simulink model "DS_distrIntp_4_0_realaxes"  (R2019b)
settings: Solver=FixedStepDiscrete  StartTime=0.0  StopTime=inf  FixedStep=Ts  RelTol=1e-3
StartFcn:
  | close all;
model workspace (MAT data in the model file):
  MvmtPerfEval_collectVal : Simulink.Parameter (value not decoded)
  MvmtPerfEval_sendOwnVal : Simulink.Parameter (value not decoded)
  PAR_center_c2 : Simulink.Parameter (value not decoded)
  PAR_numStepsAheadSmoothing : Simulink.Parameter (value not decoded)
  PAR_startPosReachedTol : Simulink.Parameter (value not decoded)
  PAR_workspace_c2 : Simulink.Parameter (value not decoded)
  PerfEval_numTicks_enable : Simulink.Parameter (value not decoded)
  Segmentregler_I_Gain : Simulink.Parameter (value not decoded)
  Segmentregler_P_Gain : Simulink.Parameter (value not decoded)
  Segmentregler_minVel_enable : Simulink.Parameter (value not decoded)
  Segmentregler_numTicks_enable : Simulink.Parameter (value not decoded)
  Ts : Simulink.Parameter (value not decoded)
  horizon : Simulink.Parameter (value not decoded)
  maxPos_x : Simulink.Parameter (value not decoded)
  maxPos_y : Simulink.Parameter (value not decoded)
  maxPos_z : Simulink.Parameter (value not decoded)
  maxVectorLengths : Simulink.Parameter (value not decoded)
  minAllowedVelSaturation : Simulink.Parameter (value not decoded)
  numAxes : Simulink.Parameter (value not decoded)
  window_length : Simulink.Parameter (value not decoded)
symbols that are objects in the model workspace (value not decoded): MvmtPerfEval_collectVal, MvmtPerfEval_sendOwnVal, numAxes, PAR_center_c2, PAR_numStepsAheadSmoothing, PAR_startPosReachedTol, PAR_workspace_c2, Ts
undefined symbols (not defined in the file or in its folder): DiscIntNeverNeededParam, setP_mat, VelOverride
libraries: vrlib x1, sldrtlib x1
(part 3 of 4)

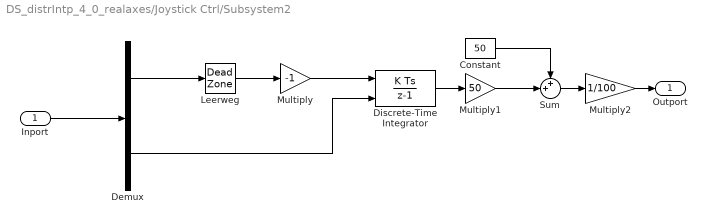
== system DS_distrIntp_4_0_realaxes/Joystick Ctrl/Subsystem2 ==
  Inport : Inport
  Constant : Constant  Value=50
  Demux : Demux  Outputs=2
  Discrete-Time Integrator : DiscreteIntegrator  gainval=0.5  ExternalReset=rising  SampleTime=-1  LimitOutput=on  UpperSaturationLimit=1  LowerSaturationLimit=-0.9  ICPrevOutput=DiscIntNeverNeededParam  ICPrevScaledInput=DiscIntNeverNeededParam
  Leerweg : DeadZone  LowerValue=-0.3  UpperValue=0.3  SaturateOnIntegerOverflow=on
  Multiply : Gain  Gain=-1
  Multiply1 : Gain  Gain=50
  Multiply2 : Gain  Gain=1/100
  Sum : Sum  Inputs=++|
  Outport : Outport  VectorParamsAs1DForOutWhenUnconnected=off
  wires:
  Multiply2/1 -> Outport/1
  Demux/2 -> Discrete-Time Integrator/2
  Demux/1 -> Leerweg/1
  Inport/1 -> Demux/1
  Sum/1 -> Multiply2/1
  Multiply1/1 -> Sum/2
  Multiply/1 -> Discrete-Time Integrator/1
  Discrete-Time Integrator/1 -> Multiply1/1
  Constant/1 -> Sum/1
  Leerweg/1 -> Multiply/1

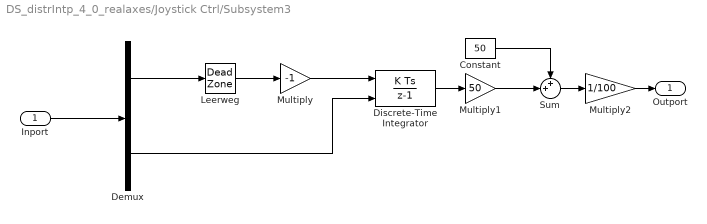
== system DS_distrIntp_4_0_realaxes/Joystick Ctrl/Subsystem3 ==
  Inport : Inport
  Constant : Constant  Value=50
  Demux : Demux  Outputs=2
  Discrete-Time Integrator : DiscreteIntegrator  gainval=0.5  ExternalReset=rising  SampleTime=-1  LimitOutput=on  UpperSaturationLimit=1  LowerSaturationLimit=-0.9  ICPrevOutput=DiscIntNeverNeededParam  ICPrevScaledInput=DiscIntNeverNeededParam
  Leerweg : DeadZone  LowerValue=-0.3  UpperValue=0.3  SaturateOnIntegerOverflow=on
  Multiply : Gain  Gain=-1
  Multiply1 : Gain  Gain=50
  Multiply2 : Gain  Gain=1/100
  Sum : Sum  Inputs=++|
  Outport : Outport  VectorParamsAs1DForOutWhenUnconnected=off
  wires:
  Leerweg/1 -> Multiply/1
  Constant/1 -> Sum/1
  Discrete-Time Integrator/1 -> Multiply1/1
  Multiply/1 -> Discrete-Time Integrator/1
  Multiply1/1 -> Sum/2
  Sum/1 -> Multiply2/1
  Inport/1 -> Demux/1
  Demux/1 -> Leerweg/1
  Demux/2 -> Discrete-Time Integrator/2
  Multiply2/1 -> Outport/1

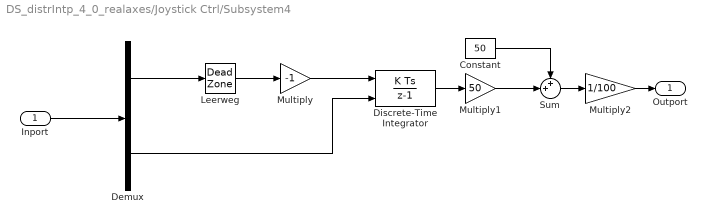
== system DS_distrIntp_4_0_realaxes/Joystick Ctrl/Subsystem4 ==
  Inport : Inport
  Constant : Constant  Value=50
  Demux : Demux  Outputs=2
  Discrete-Time Integrator : DiscreteIntegrator  gainval=0.5  ExternalReset=rising  SampleTime=-1  LimitOutput=on  UpperSaturationLimit=1  LowerSaturationLimit=-0.9  ICPrevOutput=DiscIntNeverNeededParam  ICPrevScaledInput=DiscIntNeverNeededParam
  Leerweg : DeadZone  LowerValue=-0.3  UpperValue=0.3  SaturateOnIntegerOverflow=on
  Multiply : Gain  Gain=-1
  Multiply1 : Gain  Gain=50
  Multiply2 : Gain  Gain=1/100
  Sum : Sum  Inputs=++|
  Outport : Outport  VectorParamsAs1DForOutWhenUnconnected=off
  wires:
  Leerweg/1 -> Multiply/1
  Constant/1 -> Sum/1
  Discrete-Time Integrator/1 -> Multiply1/1
  Multiply/1 -> Discrete-Time Integrator/1
  Multiply1/1 -> Sum/2
  Sum/1 -> Multiply2/1
  Inport/1 -> Demux/1
  Demux/1 -> Leerweg/1
  Demux/2 -> Discrete-Time Integrator/2
  Multiply2/1 -> Outport/1

== stateflow chart DS_distrIntp_4_0_realaxes/Coordination ==
  state funcs [group]
  state Dispatcher [parallel]
    settings: executionOrder=1
    state Idle
    state Registriere_Achse
      entry: num_registeredAxes = ...
      num_registeredAxes + 1;
    state Erhalte_Koordinationsvektor
      entry:
      num_collectedCVectors = ...
      num_collectedCVectors + 1;
      cVectors = [cVectors; cVector_exchange];
      FLAG_canSend_cVector = 1;
    state Distribute_Coordination_Info
      entry:
      FLAG_cVectors_complete = 1;
    state Registriere_Achsen_bereit
      entry:
      num_readyAxes = num_readyAxes + daten;
      if(num_readyAxes == 16)
      FLAG_allAxesReady = true;
      num_readyAxes = 0;
      end
    state axis_run_counter
      entry:
      num_runningAxes = num_runningAxes + daten;
      if num_runningAxes == 16
      FLAG_startButton = false;
      FLAG_axesRunning = true;
      FLAG_allAxesReady = false;
      end
    state axis_stop_counter
      entry:
      num_runningAxes = num_runningAxes - daten;
      if(num_runningAxes == 0)
      FLAG_stopButton = false;
      FLAG_axesRunning = false;
      end
    state DONE
      entry:
      num_doneAxes = num_doneAxes + 1;
      if num_doneAxes == num_registeredAxes
      %FLAG_stopSim = 1;
      end
    state Movement_Performance_Evaluation
      entry:
      while receive(MvmtPerfCoeff)
      if MvmtPerfCoeff.data > MvmtPerf
      MvmtPerf = MvmtPerfCoeff.data;
      end
      if MvmtPerfCoeff.data == -1
      MvmtPerf = 1;
      end
      discard(MvmtPerfCoeff);
      end
    (default) -> Idle
    Idle -> Registriere_Achse [order 1] : registerAxis
    Registriere_Achse -> Idle
    Idle -> Erhalte_Koordinationsvektor [order 2] : cVector_sent
    Erhalte_Koordinationsvektor -> Idle
    Idle -> Distribute_Coordination_Info [order 3] : [num_collectedCVectors==...
        | num_registeredAxes && ...
        | FLAG_cVectors_complete == 0]
    Distribute_Coordination_Info -> Idle
    Idle -> Registriere_Achsen_bereit [order 4] : axis_ready{daten=axis_ready.data}
    Registriere_Achsen_bereit -> Idle
    Idle -> axis_run_counter [order 5] : axis_isRunning{daten=axis_isRunning.data}
    axis_run_counter -> Idle
    Idle -> axis_stop_counter [order 8] : axis_isNotRunning{daten=axis_isNotRunning.data}
    axis_stop_counter -> Idle
    Idle -> Dispatcher.DONE [order 6] : axis_done
    Dispatcher.DONE -> Idle
    Idle -> Movement_Performance_Evaluation [order 7] : MvmtPerfCoeff
    Movement_Performance_Evaluation -> Idle
  state Axis_X [parallel]
    settings: executionOrder=2
    state Start_Idle
      entry:
      registerAxis.data = true;
      send(registerAxis)
    state Hermite_Interpolation
      entry:
      if FLAG_doAkima == 1
      iP = funcs.DS_hermIntp(setP,setP_dist);
      else
      iP = setP;
      end
    state Koordinationsvektor
      entry:
      cVector_init = funcs.DS_gen_Cvector_init...
      (iP,PAR_isAxis,PAR_maxVel);
    state Koordinationsvektor_austauschen
      during:
      if FLAG_canSend_cVector == 1
      cVector_exchange = cVector_init;
      FLAG_canSend_cVector = 0;
      send(cVector_sent);
      axisHasSentCVector = 1;
      end
      Axis_X.Koordinationsvektor_austauschen -> Axis_X.Koordinationsvektor_austauschen [order 1]
    state Axis_full_reset
      state JogAxis
        entry:
        ResetAxis(PAR_isAxis);
        currPos = GET_istPos(PAR_isAxis,1);
        jogAxis(PAR_isAxis);
      state Check_if_moving
        entry:
        %jogAxis(PAR_isAxis);
        if(abs(currPos - GET_istPos(PAR_isAxis,1)) > ...
        PAR_resetAxis_deltaS)
        axis_is_moving = 1;
        else
        axis_is_moving = 0;
        end
      state Reset_successful
        entry:
        jogAxis(PAR_isAxis);
        axis_is_moving = 0;
        FLAG_resetAxis(PAR_isAxis) = 0;
      (default) -> Axis_X.Axis_full_reset.JogAxis
      Axis_X.Axis_full_reset.JogAxis -> Axis_X.Axis_full_reset.Check_if_moving : after(2,'sec')
      Axis_X.Axis_full_reset.Check_if_moving -> Axis_X.Axis_full_reset.JogAxis [order 2] : [axis_is_moving == 0]
      Axis_X.Axis_full_reset.Check_if_moving -> Axis_X.Axis_full_reset.Reset_successful [order 1] : [axis_is_moving == 1]
    state Wait_for_cVectors
    state Find_Consensus
      entry: execVec = funcs.DS_find_Consensus(iP,cVectors,...
      PAR_execIteratorStepSize,PAR_isAxis);
    state Axis_ok
      state Bootstrap_MotionControl
        state JogAxis
          entry:
          ff = ff + 1;
          FLAG_bootstrap_completed = 0;
          %ResetAxis(PAR_isAxis);
          moveRel(PAR_isAxis,PAR_Bootstrap_deltaS,PAR_maxVel/10);
        state GoToStartPos
          entry:
          goToPos(PAR_isAxis,setP(PAR_isAxis,1)*1000,PAR_maxVel*0.5);
        state Check_StartPos_reached
          during:
          if(abs(GET_istPos(PAR_isAxis,1) - setP(PAR_isAxis,1)) <...
          PAR_startPosReachedTol)
          FLAG_bootstrap_completed = 1;
          end
        state StartPos_reached
          entry:
          %on after(3,sec):
          axis_ready.data = 1;
          send(axis_ready);
        (default) -> Axis_X.Axis_ok.Bootstrap_MotionControl.JogAxis
        Axis_X.Axis_ok.Bootstrap_MotionControl.JogAxis -> Axis_X.Axis_ok.Bootstrap_MotionControl.GoToStartPos : after(1,'sec')
        Axis_X.Axis_ok.Bootstrap_MotionControl.GoToStartPos -> Axis_X.Axis_ok.Bootstrap_MotionControl.Check_StartPos_reached
        Axis_X.Axis_ok.Bootstrap_MotionControl.Check_StartPos_reached -> Axis_X.Axis_ok.Bootstrap_MotionControl.StartPos_reached : after(5,sec)[FLAG_bootstrap_completed == 1]
      state Start_run
        entry:
        axis_isRunning.data = 1;
        send(axis_isRunning);
        RUN_idx = 0;
        RUN_startPos(1,PAR_isAxis) = setP(PAR_isAxis,1);
        RUN_num_steps = size(execVec,2);
        state Send_command
          entry:
          RUN_idx = RUN_idx + 1;
          currCVector = cVectors(:,RUN_idx)' ./ VelOverride';
          currCVal = max(currCVector);
          currOverrideAdaptationFactor = execVec(3,RUN_idx) / currCVal; %individueller neuer Override Faktor für diese Achse
          currStepTimeLength = execVec(3,RUN_idx) / currOverrideAdaptationFactor;
          RUN_pos(1,PAR_isAxis) = execVec(1,RUN_idx);
          RUN_vel(1,PAR_isAxis) = execVec(2,RUN_idx) * currOverrideAdaptationFactor;
          MvmtPerf_accumulatedLagTime = MvmtPerf_accumulatedLagTime + (currStepTimeLength - execVec(3,RUN_idx));
          RUN_time(1,PAR_isAxis) = execVec(4,RUN_idx) + MvmtPerf_accumulatedLagTime; %wird nicht benutzt
          RUN_maxVel(1,PAR_isAxis) = PAR_maxVel;
          RUN_MvmtPerfFeedback(1,PAR_isAxis) = 0; %wird zZt nicht benutzt
        state execute_movement
          state DEVEKOS_Ueberschleifen
            entry:
            currStepTimeLength = currStepTimeLength - PAR_numStepsAheadSmoothing*Ts;
          state idle
            entry:
            MvmtPerfCoeff.data = -1;
            send(MvmtPerfCoeff);
          state getOwnPerfCoeff [commented out]
            entry:
            MvmtPerfCoeff.data = GET_perfIndicator(PAR_isAxis);
            send(MvmtPerfCoeff);
          state getMutualPerformance [commented out]
            entry:
            MvmtPerf_accumulatedLagTime = MvmtPerf_accumulatedLagTime + (MvmtPerf-1) * currStepTimeLength;
            RUN_MvmtPerfFeedback(1,PAR_isAxis) = (MvmtPerf-1) * currStepTimeLength;
            RUN_vel(1,PAR_isAxis) = execVec(2,RUN_idx) / MvmtPerf;
            currStepTimeLength = currStepTimeLength * MvmtPerf;
          (default) -> Axis_X.Axis_ok.Start_run.execute_movement.idle
          Axis_X.Axis_ok.Start_run.execute_movement.idle -> Axis_X.Axis_ok.Start_run.execute_movement.DEVEKOS_Ueberschleifen
          Axis_X.Axis_ok.Start_run.execute_movement.idle -> Axis_X.Axis_ok.Start_run.execute_movement.getOwnPerfCoeff [commented out] : after(currStepTimeLength * MvmtPerfEval_sendOwnVal,sec)
          Axis_X.Axis_ok.Start_run.execute_movement.getOwnPerfCoeff -> Axis_X.Axis_ok.Start_run.execute_movement.getMutualPerformance [commented out] : after(currStepTimeLength * (MvmtPerfEval_collectVal - MvmtPerfEval_sendOwnVal),sec)
        (default) -> Axis_X.Axis_ok.Start_run.Send_command
        (junction 638) -> Axis_X.Axis_ok.Start_run.Send_command [order 2]
        Axis_X.Axis_ok.Start_run.Send_command -> Axis_X.Axis_ok.Start_run.execute_movement
        Axis_X.Axis_ok.Start_run.execute_movement -> (junction 638) : after(currStepTimeLength,sec)
      (junction 2099) -> (junction 1942)
      (junction 1947) -> (junction 2099)
      (junction 1942) -> Axis_X.Axis_ok.Bootstrap_MotionControl
      Axis_X.Axis_ok.Bootstrap_MotionControl -> Axis_X.Axis_ok.Start_run [order 2] : [FLAG_allAxesReady == 1 &&...
          |  FLAG_startButton == 1]
      Axis_X.Axis_ok.Bootstrap_MotionControl -> Axis_X.Axis_ok.Start_run [order 1] : [FLAG_allAxesReady == 1 &&...
          |  FLAG_runContinuously == 1]
      Axis_X.Axis_ok.Start_run -> (junction 1947) : [FLAG_stopButton == 1]...
          | {StopAxis(PAR_isAxis);...
          | axis_isNotRunning.data = 1;...
          | send(axis_isNotRunning)}
    state DONE
      entry:
      StopAxis(PAR_isAxis);
      %send(axis_isNotRunning);
      %send(axis_done);
      exit:
      axis_isNotRunning.data = 1;
      send(axis_isNotRunning);
    (default) -> Axis_X.Start_Idle
    Axis_X.Start_Idle -> Axis_X.Hermite_Interpolation
    Axis_X.Hermite_Interpolation -> Axis_X.Koordinationsvektor
    Axis_X.Koordinationsvektor -> Axis_X.Koordinationsvektor_austauschen
    Axis_X.Koordinationsvektor_austauschen -> Axis_X.Wait_for_cVectors [order 1] : [axisHasSentCVector == 1]
    Axis_X.Wait_for_cVectors -> Axis_X.Find_Consensus : [FLAG_cVectors_complete == 1]
    Axis_X.Axis_full_reset -> (junction 2110) : [FLAG_resetAxis(PAR_isAxis) == 0]
    Axis_X.Axis_ok -> Axis_X.Axis_full_reset : [FLAG_resetAxis(PAR_isAxis) == 1]...
        | {StopAxis(PAR_isAxis);...
        | axis_isNotRunning.data = 1;...
        | send(axis_isNotRunning)}
    Axis_X.Find_Consensus -> (junction 2103)
    (junction 2110) -> (junction 2103)
    (junction 2103) -> (junction 1942)
    (junction 2388) -> (junction 1947)
    (junction 638) -> Axis_X.DONE [order 1] : [RUN_idx == RUN_num_steps]
    Axis_X.DONE -> (junction 2388)
  state Axis_Y [parallel]
    settings: executionOrder=3
    state Start_Idle
      entry:
      registerAxis.data = true;
      send(registerAxis)
    state Hermite_Interpolation
      entry:
      if FLAG_doAkima == 1
      iP = funcs.DS_hermIntp(setP,setP_dist);
      else
      iP = setP;
      end
    state Koordinationsvektor
      entry:
      cVector_init = funcs.DS_gen_Cvector_init...
      (iP,PAR_isAxis,PAR_maxVel);
    state Koordinationsvektor_austauschen
      during:
      if FLAG_canSend_cVector == 1
      cVector_exchange = cVector_init;
      FLAG_canSend_cVector = 0;
      send(cVector_sent);
      axisHasSentCVector = 1;
      end
      Axis_Y.Koordinationsvektor_austauschen -> Axis_Y.Koordinationsvektor_austauschen [order 1]
    state Axis_full_reset
      state JogAxis
        entry:
        ResetAxis(PAR_isAxis);
        currPos = GET_istPos(PAR_isAxis,1);
        jogAxis(PAR_isAxis);
      state Check_if_moving
        entry:
        %jogAxis(PAR_isAxis);
        if(abs(currPos - GET_istPos(PAR_isAxis,1)) > ...
        PAR_resetAxis_deltaS)
        axis_is_moving = 1;
        else
        axis_is_moving = 0;
        end
      state Reset_successful
        entry:
        jogAxis(PAR_isAxis);
        axis_is_moving = 0;
        FLAG_resetAxis(PAR_isAxis) = 0;
      (default) -> Axis_Y.Axis_full_reset.JogAxis
      Axis_Y.Axis_full_reset.JogAxis -> Axis_Y.Axis_full_reset.Check_if_moving : after(2,'sec')
      Axis_Y.Axis_full_reset.Check_if_moving -> Axis_Y.Axis_full_reset.JogAxis [order 2] : [axis_is_moving == 0]
      Axis_Y.Axis_full_reset.Check_if_moving -> Axis_Y.Axis_full_reset.Reset_successful [order 1] : [axis_is_moving == 1]
    state Wait_for_cVectors
    state Find_Consensus
      entry: execVec = funcs.DS_find_Consensus(iP,cVectors,...
      PAR_execIteratorStepSize,PAR_isAxis);
      ff = 1;
    state Axis_ok
      state Bootstrap_MotionControl
        state JogAxis
          entry:
          FLAG_bootstrap_completed = 0;
          ResetAxis(PAR_isAxis);
          moveRel(PAR_isAxis,PAR_Bootstrap_deltaS,PAR_maxVel/10);
        state GoToStartPos
          entry:
          goToPos(PAR_isAxis,setP(PAR_isAxis,1)*1000,PAR_maxVel*0.5);
        state Check_StartPos_reached
          during:
          if(abs(GET_istPos(PAR_isAxis,1) - setP(PAR_isAxis,1)) <...
          PAR_startPosReachedTol)
          FLAG_bootstrap_completed = 1;
          end
        state StartPos_reached
          entry:
          %on after(3,sec):
          axis_ready.data = 3;
          send(axis_ready);
        (default) -> Axis_Y.Axis_ok.Bootstrap_MotionControl.JogAxis
        Axis_Y.Axis_ok.Bootstrap_MotionControl.JogAxis -> Axis_Y.Axis_ok.Bootstrap_MotionControl.GoToStartPos : after(1,'sec')
        Axis_Y.Axis_ok.Bootstrap_MotionControl.GoToStartPos -> Axis_Y.Axis_ok.Bootstrap_MotionControl.Check_StartPos_reached
        Axis_Y.Axis_ok.Bootstrap_MotionControl.Check_StartPos_reached -> Axis_Y.Axis_ok.Bootstrap_MotionControl.StartPos_reached : [FLAG_bootstrap_completed == 1]
      state Start_run
        entry:
        axis_isRunning.data = 3;
        send(axis_isRunning);
        RUN_idx = 0;
        RUN_startPos(1,PAR_isAxis) = setP(PAR_isAxis,1);
        RUN_num_steps = size(execVec,2);
        state Send_command
          entry:
          RUN_idx = RUN_idx + 1;
          currCVector = cVectors(:,RUN_idx)' ./ VelOverride';
          currCVal = max(currCVector);
          currOverrideAdaptationFactor = execVec(3,RUN_idx) / currCVal; %individueller neuer Override Faktor für diese Achse
          currStepTimeLength = execVec(3,RUN_idx) / currOverrideAdaptationFactor;
          RUN_pos(1,PAR_isAxis) = execVec(1,RUN_idx);
          RUN_vel(1,PAR_isAxis) = execVec(2,RUN_idx) * currOverrideAdaptationFactor;
          MvmtPerf_accumulatedLagTime = MvmtPerf_accumulatedLagTime + (currStepTimeLength - execVec(3,RUN_idx));
          RUN_time(1,PAR_isAxis) = execVec(4,RUN_idx) + MvmtPerf_accumulatedLagTime; %wird nicht benutzt
          RUN_maxVel(1,PAR_isAxis) = PAR_maxVel;
          RUN_MvmtPerfFeedback(1,PAR_isAxis) = 0; %wird zZt nicht benutzt
        state execute_movement
          state DEVEKOS_Ueberschleifen
            entry:
            currStepTimeLength = currStepTimeLength - PAR_numStepsAheadSmoothing*Ts;
          state idle
            entry:
            MvmtPerfCoeff.data = -1;
            send(MvmtPerfCoeff);
          state getOwnPerfCoeff [commented out]
            entry:
            MvmtPerfCoeff.data = GET_perfIndicator(PAR_isAxis);
            send(MvmtPerfCoeff);
          state getMutualPerformance [commented out]
            entry:
            MvmtPerf_accumulatedLagTime = MvmtPerf_accumulatedLagTime + (MvmtPerf-1) * currStepTimeLength;
            RUN_MvmtPerfFeedback(1,PAR_isAxis) = (MvmtPerf-1) * currStepTimeLength;
            RUN_vel(1,PAR_isAxis) = execVec(2,RUN_idx) / MvmtPerf;
            currStepTimeLength = currStepTimeLength * MvmtPerf;
          (default) -> Axis_Y.Axis_ok.Start_run.execute_movement.idle
          Axis_Y.Axis_ok.Start_run.execute_movement.idle -> Axis_Y.Axis_ok.Start_run.execute_movement.DEVEKOS_Ueberschleifen
          Axis_Y.Axis_ok.Start_run.execute_movement.idle -> Axis_Y.Axis_ok.Start_run.execute_movement.getOwnPerfCoeff [commented out] : after(currStepTimeLength * MvmtPerfEval_sendOwnVal,sec)
          Axis_Y.Axis_ok.Start_run.execute_movement.getOwnPerfCoeff -> Axis_Y.Axis_ok.Start_run.execute_movement.getMutualPerformance [commented out] : after(currStepTimeLength * (MvmtPerfEval_collectVal - MvmtPerfEval_sendOwnVal),sec)
        (default) -> Axis_Y.Axis_ok.Start_run.Send_command
        (junction 2720) -> Axis_Y.Axis_ok.Start_run.Send_command [order 2]
        Axis_Y.Axis_ok.Start_run.Send_command -> Axis_Y.Axis_ok.Start_run.execute_movement
        Axis_Y.Axis_ok.Start_run.execute_movement -> (junction 2720) : after(currStepTimeLength,sec)
      (junction 2700) -> (junction 2699)
      (junction 2701) -> (junction 2700)
      (junction 2699) -> Axis_Y.Axis_ok.Bootstrap_MotionControl
      Axis_Y.Axis_ok.Bootstrap_MotionControl -> Axis_Y.Axis_ok.Start_run [order 2] : [FLAG_allAxesReady == 1 &&...
          |  FLAG_startButton == 1]
      Axis_Y.Axis_ok.Bootstrap_MotionControl -> Axis_Y.Axis_ok.Start_run [order 1] : [FLAG_allAxesReady == 1 &&...
          |  FLAG_runContinuously == 1]
      Axis_Y.Axis_ok.Start_run -> (junction 2701) : [FLAG_stopButton == 1]...
          | {StopAxis(PAR_isAxis);...
          | axis_isNotRunning.data = 3;...
          | send(axis_isNotRunning)}
    state DONE
      entry:
      StopAxis(PAR_isAxis);
      %send(axis_done);
      exit:
      axis_isNotRunning.data = 3;
      send(axis_isNotRunning);
    (default) -> Axis_Y.Start_Idle
    Axis_Y.Start_Idle -> Axis_Y.Hermite_Interpolation
    Axis_Y.Hermite_Interpolation -> Axis_Y.Koordinationsvektor
    Axis_Y.Koordinationsvektor -> Axis_Y.Koordinationsvektor_austauschen
    Axis_Y.Koordinationsvektor_austauschen -> Axis_Y.Wait_for_cVectors [order 1] : [axisHasSentCVector == 1]
    Axis_Y.Wait_for_cVectors -> Axis_Y.Find_Consensus : [FLAG_cVectors_complete == 1]
    Axis_Y.Axis_full_reset -> (junction 2651) : [FLAG_resetAxis(PAR_isAxis) == 0]
    Axis_Y.Axis_ok -> Axis_Y.Axis_full_reset : [FLAG_resetAxis(PAR_isAxis) == 1]...
        | {StopAxis(PAR_isAxis);...
        | axis_isNotRunning.data = 3;...
        | send(axis_isNotRunning)}
    Axis_Y.Find_Consensus -> (junction 2650)
    (junction 2651) -> (junction 2650)
    (junction 2650) -> (junction 2699)
    (junction 2652) -> (junction 2701)
    (junction 2720) -> Axis_Y.DONE [order 1] : [RUN_idx == RUN_num_steps]
    Axis_Y.DONE -> (junction 2652)
  state Axis_Z [parallel]
    settings: executionOrder=4
    state Start_Idle
      entry:
      registerAxis.data = true;
      send(registerAxis)
    state Hermite_Interpolation
      entry:
      if FLAG_doAkima == 1
      iP = funcs.DS_hermIntp(setP,setP_dist);
      else
      iP = setP;
      end
    state Koordinationsvektor
      entry:
      cVector_init = funcs.DS_gen_Cvector_init...
      (iP,PAR_isAxis,PAR_maxVel);
    state Koordinationsvektor_austauschen
      during:
      if FLAG_canSend_cVector == 1
      cVector_exchange = cVector_init;
      FLAG_canSend_cVector = 0;
      send(cVector_sent);
      axisHasSentCVector = 1;
      end
      Axis_Z.Koordinationsvektor_austauschen -> Axis_Z.Koordinationsvektor_austauschen [order 1]
    state Axis_full_reset
      state JogAxis
        entry:
        ResetAxis(PAR_isAxis);
        currPos = GET_istPos(PAR_isAxis,1);
        jogAxis(PAR_isAxis);
      state Check_if_moving
        entry:
        %jogAxis(PAR_isAxis);
        if(abs(currPos - GET_istPos(PAR_isAxis,1)) > ...
        PAR_resetAxis_deltaS)
        axis_is_moving = 1;
        else
        axis_is_moving = 0;
        end
      state Reset_successful
        entry:
        jogAxis(PAR_isAxis);
        axis_is_moving = 0;
        FLAG_resetAxis(PAR_isAxis) = 0;
      (default) -> Axis_Z.Axis_full_reset.JogAxis
      Axis_Z.Axis_full_reset.JogAxis -> Axis_Z.Axis_full_reset.Check_if_moving : after(2,'sec')
      Axis_Z.Axis_full_reset.Check_if_moving -> Axis_Z.Axis_full_reset.JogAxis [order 2] : [axis_is_moving == 0]
      Axis_Z.Axis_full_reset.Check_if_moving -> Axis_Z.Axis_full_reset.Reset_successful [order 1] : [axis_is_moving == 1]
    state Wait_for_cVectors
    state Find_Consensus
      entry: execVec = funcs.DS_find_Consensus(iP,cVectors,...
      PAR_execIteratorStepSize,PAR_isAxis);
    state Axis_ok
      state Bootstrap_MotionControl
        state JogAxis
          entry:
          FLAG_bootstrap_completed = 0;
          ResetAxis(PAR_isAxis);
          moveRel(PAR_isAxis,PAR_Bootstrap_deltaS,PAR_maxVel/10);
        state GoToStartPos
          entry:
          goToPos(PAR_isAxis,setP(PAR_isAxis,1)*1000,PAR_maxVel*0.5);
        state Check_StartPos_reached
          during:
          if(abs(GET_istPos(PAR_isAxis,1) - setP(PAR_isAxis,1)) <...
          PAR_startPosReachedTol)
          FLAG_bootstrap_completed = 1;
          end
        state StartPos_reached
          entry:
          axis_ready.data = 5;
          send(axis_ready);
        (default) -> Axis_Z.Axis_ok.Bootstrap_MotionControl.JogAxis
        Axis_Z.Axis_ok.Bootstrap_MotionControl.JogAxis -> Axis_Z.Axis_ok.Bootstrap_MotionControl.GoToStartPos : after(1,'sec')
        Axis_Z.Axis_ok.Bootstrap_MotionControl.GoToStartPos -> Axis_Z.Axis_ok.Bootstrap_MotionControl.Check_StartPos_reached
        Axis_Z.Axis_ok.Bootstrap_MotionControl.Check_StartPos_reached -> Axis_Z.Axis_ok.Bootstrap_MotionControl.StartPos_reached : [FLAG_bootstrap_completed == 1]
      state Start_run
        entry:
        axis_isRunning.data = 5;
        send(axis_isRunning);
        RUN_idx = 0;
        RUN_startPos(1,PAR_isAxis) = setP(PAR_isAxis,1);
        RUN_num_steps = size(execVec,2);
        state Send_command
          entry:
          RUN_idx = RUN_idx + 1;
          currCVector = cVectors(:,RUN_idx)' ./ VelOverride';
          currCVal = max(currCVector);
          currOverrideAdaptationFactor = execVec(3,RUN_idx) / currCVal; %individueller neuer Override Faktor für diese Achse
          currStepTimeLength = execVec(3,RUN_idx) / currOverrideAdaptationFactor;
          RUN_pos(1,PAR_isAxis) = execVec(1,RUN_idx);
          RUN_vel(1,PAR_isAxis) = execVec(2,RUN_idx) * currOverrideAdaptationFactor;
          MvmtPerf_accumulatedLagTime = MvmtPerf_accumulatedLagTime + (currStepTimeLength - execVec(3,RUN_idx));
          RUN_time(1,PAR_isAxis) = execVec(4,RUN_idx) + MvmtPerf_accumulatedLagTime; %wird nicht benutzt
          RUN_maxVel(1,PAR_isAxis) = PAR_maxVel;
          RUN_MvmtPerfFeedback(1,PAR_isAxis) = 0; %wird zZt nicht benutzt
        state execute_movement
          state DEVEKOS_Ueberschleifen
            entry:
            currStepTimeLength = currStepTimeLength - PAR_numStepsAheadSmoothing*Ts;
          state idle
            entry:
            MvmtPerfCoeff.data = -1;
            send(MvmtPerfCoeff);
          state getOwnPerfCoeff [commented out]
            entry:
            MvmtPerfCoeff.data = GET_perfIndicator(PAR_isAxis);
            send(MvmtPerfCoeff);
          state getMutualPerformance [commented out]
            entry:
            MvmtPerf_accumulatedLagTime = MvmtPerf_accumulatedLagTime + (MvmtPerf-1) * currStepTimeLength;
            RUN_MvmtPerfFeedback(1,PAR_isAxis) = (MvmtPerf-1) * currStepTimeLength;
            RUN_vel(1,PAR_isAxis) = execVec(2,RUN_idx) / MvmtPerf;
            currStepTimeLength = currStepTimeLength * MvmtPerf;
          (default) -> Axis_Z.Axis_ok.Start_run.execute_movement.idle
          Axis_Z.Axis_ok.Start_run.execute_movement.idle -> Axis_Z.Axis_ok.Start_run.execute_movement.DEVEKOS_Ueberschleifen
          Axis_Z.Axis_ok.Start_run.execute_movement.idle -> Axis_Z.Axis_ok.Start_run.execute_movement.getOwnPerfCoeff [commented out] : after(currStepTimeLength * MvmtPerfEval_sendOwnVal,sec)
          Axis_Z.Axis_ok.Start_run.execute_movement.getOwnPerfCoeff -> Axis_Z.Axis_ok.Start_run.execute_movement.getMutualPerformance [commented out] : after(currStepTimeLength * (MvmtPerfEval_collectVal - MvmtPerfEval_sendOwnVal),sec)
        (default) -> Axis_Z.Axis_ok.Start_run.Send_command
        (junction 2823) -> Axis_Z.Axis_ok.Start_run.Send_command [order 2]
        Axis_Z.Axis_ok.Start_run.Send_command -> Axis_Z.Axis_ok.Start_run.execute_movement
        Axis_Z.Axis_ok.Start_run.execute_movement -> (junction 2823) : after(currStepTimeLength,sec)
      (junction 2803) -> (junction 2802)
      (junction 2804) -> (junction 2803)
      (junction 2802) -> Axis_Z.Axis_ok.Bootstrap_MotionControl
      Axis_Z.Axis_ok.Bootstrap_MotionControl -> Axis_Z.Axis_ok.Start_run [order 2] : [FLAG_allAxesReady == 1 &&...
          |  FLAG_startButton == 1]
      Axis_Z.Axis_ok.Bootstrap_MotionControl -> Axis_Z.Axis_ok.Start_run [order 1] : [FLAG_allAxesReady == 1 &&...
          |  FLAG_runContinuously == 1]
      Axis_Z.Axis_ok.Start_run -> (junction 2804) : [FLAG_stopButton == 1]...
          | {StopAxis(PAR_isAxis);...
          | axis_isNotRunning.data = 5;...
          | send(axis_isNotRunning)}
    state DONE
      entry:
      StopAxis(PAR_isAxis);
      %send(axis_done);
      exit:
      axis_isNotRunning.data = 5;
      send(axis_isNotRunning);
    (default) -> Axis_Z.Start_Idle
    Axis_Z.Start_Idle -> Axis_Z.Hermite_Interpolation
    Axis_Z.Hermite_Interpolation -> Axis_Z.Koordinationsvektor
    Axis_Z.Koordinationsvektor -> Axis_Z.Koordinationsvektor_austauschen
    Axis_Z.Koordinationsvektor_austauschen -> Axis_Z.Wait_for_cVectors [order 1] : [axisHasSentCVector == 1]
    Axis_Z.Wait_for_cVectors -> Axis_Z.Find_Consensus : [FLAG_cVectors_complete == 1]
    Axis_Z.Axis_full_reset -> (junction 2754) : [FLAG_resetAxis(PAR_isAxis) == 0]
    Axis_Z.Axis_ok -> Axis_Z.Axis_full_reset : [FLAG_resetAxis(PAR_isAxis) == 1]...
        | {StopAxis(PAR_isAxis);...
        | axis_isNotRunning.data = 5;...
        | send(axis_isNotRunning)}
    Axis_Z.Find_Consensus -> (junction 2753)
    (junction 2754) -> (junction 2753)
    (junction 2753) -> (junction 2802)
    (junction 2755) -> (junction 2804)
    (junction 2823) -> Axis_Z.DONE [order 1] : [RUN_idx == RUN_num_steps]
    Axis_Z.DONE -> (junction 2755)
  state Axis_C2 [parallel]
    settings: executionOrder=5
    state Start_Idle
      entry:
      registerAxis.data = true;
      send(registerAxis)
    state Bahnpunkte
      entry:
      if FLAG_doAkima == 1
      iP = funcs.DS_hermIntp(setP,setP_dist);
      else
      iP = setP;
      end
      if PAR_isAxis > 3
      iP = [iP;zeros(PAR_isAxis - size(iP,1), length(iP))];
      iP(PAR_isAxis,:) = funcs.PS_gen_Points_Axis...
      (iP,PAR_center_c2,...
      PAR_workspace_c2,...
      PAR_kindOfAxis);
      end
    state Koordinationsvektor
      entry:
      cVector_init = funcs.DS_gen_Cvector_init...
      (iP,PAR_isAxis,PAR_maxVel);
    state Koordinationsvektor_austauschen
      during:
      if FLAG_canSend_cVector == 1
      cVector_exchange = cVector_init;
      FLAG_canSend_cVector = 0;
      send(cVector_sent);
      axisHasSentCVector = 1;
      end
      Axis_C2.Koordinationsvektor_austauschen -> Axis_C2.Koordinationsvektor_austauschen [order 1]
    state Wait_for_cVectors
    state Find_Consensus
      entry:
      execVec = funcs.DS_find_Consensus(iP,cVectors,...
      PAR_execIteratorStepSize,PAR_isAxis);
      axis_ready.data = 7;
      send(axis_ready);
    state Nullen
      entry:
      homingDauerlauf;
    state Homing_done
      entry:
      axis_ready.data = 7;
      send(axis_ready);
    state Start_run
      entry:
      axis_isRunning.data = 7;
      send(axis_isRunning);
      RUN_idx = 0;
      RUN_startPos(1,PAR_isAxis) = iP(PAR_isAxis,1);
      RUN_num_steps = size(execVec,2);
      state Send_command
        entry:
        RUN_idx = RUN_idx + 1;
        currCVector = cVectors(:,RUN_idx)' ./ VelOverride';
        currCVal = max(currCVector);
        currOverrideAdaptationFactor = execVec(3,RUN_idx) / currCVal; %individueller neuer Override Faktor für diese Achse
        currStepTimeLength = execVec(3,RUN_idx) / currOverrideAdaptationFactor;
        RUN_pos(1,PAR_isAxis) = execVec(1,RUN_idx);
        RUN_vel(1,PAR_isAxis) = execVec(2,RUN_idx) * currOverrideAdaptationFactor;
        MvmtPerf_accumulatedLagTime = MvmtPerf_accumulatedLagTime + (currStepTimeLength - execVec(3,RUN_idx));
        RUN_time(1,PAR_isAxis) = execVec(4,RUN_idx) + MvmtPerf_accumulatedLagTime; %wird nicht benutzt
        RUN_maxVel(1,PAR_isAxis) = PAR_maxVel;
        RUN_MvmtPerfFeedback(1,PAR_isAxis) = 0; %wird zZt nicht benutzt
      state execute_movement
        state DEVEKOS_Ueberschleifen
          entry:
          currStepTimeLength = currStepTimeLength - PAR_numStepsAheadSmoothing*Ts;
        state idle
          entry:
          MvmtPerfCoeff.data = -1;
          send(MvmtPerfCoeff);
        state getOwnPerfCoeff [commented out]
          entry:
          MvmtPerfCoeff.data = GET_perfIndicator(PAR_isAxis);
          send(MvmtPerfCoeff);
        state getMutualPerformance [commented out]
          entry:
          MvmtPerf_accumulatedLagTime = MvmtPerf_accumulatedLagTime + (MvmtPerf-1) * currStepTimeLength;
          RUN_MvmtPerfFeedback(1,PAR_isAxis) = (MvmtPerf-1) * currStepTimeLength;
          RUN_vel(1,PAR_isAxis) = execVec(2,RUN_idx) / MvmtPerf;
          currStepTimeLength = currStepTimeLength * MvmtPerf;
        (default) -> Axis_C2.Start_run.execute_movement.idle
        Axis_C2.Start_run.execute_movement.idle -> Axis_C2.Start_run.execute_movement.DEVEKOS_Ueberschleifen
        Axis_C2.Start_run.execute_movement.idle -> Axis_C2.Start_run.execute_movement.getOwnPerfCoeff [commented out] : after(currStepTimeLength * MvmtPerfEval_sendOwnVal,sec)
        Axis_C2.Start_run.execute_movement.getOwnPerfCoeff -> Axis_C2.Start_run.execute_movement.getMutualPerformance [commented out] : after(currStepTimeLength * (MvmtPerfEval_collectVal - MvmtPerfEval_sendOwnVal),sec)
      (default) -> Axis_C2.Start_run.Send_command
      (junction 2372) -> Axis_C2.Start_run.Send_command [order 2]
      Axis_C2.Start_run.Send_command -> Axis_C2.Start_run.execute_movement
      Axis_C2.Start_run.execute_movement -> (junction 2372) : after(currStepTimeLength,sec)
    state DONE
      entry:
      %send(axis_done);
      exit:
      axis_isNotRunning.data = 7;
      send(axis_isNotRunning);
    (default) -> Axis_C2.Start_Idle
    Axis_C2.Start_Idle -> Bahnpunkte
    Bahnpunkte -> Axis_C2.Koordinationsvektor
    Axis_C2.Koordinationsvektor -> Axis_C2.Koordinationsvektor_austauschen
    Axis_C2.Koordinationsvektor_austauschen -> Axis_C2.Wait_for_cVectors [order 1] : [axisHasSentCVector == 1]
    Axis_C2.Wait_for_cVectors -> Axis_C2.Find_Consensus : [FLAG_cVectors_complete == 1]
    Axis_C2.Find_Consensus -> (junction 2595)
    Nullen -> Homing_done : after(3,sec)
    (junction 2628) -> Nullen
    Homing_done -> (junction 2595)
    (junction 2595) -> Axis_C2.Start_run [order 1] : [FLAG_allAxesReady == 1 &&...
        |  FLAG_startButton == 1]
    (junction 2595) -> Axis_C2.Start_run [order 2] : [FLAG_allAxesReady == 1 &&...
        |  FLAG_runContinuously == 1]
    Axis_C2.Start_run -> (junction 2628) : [FLAG_stopButton == 1]...
        | {axis_isNotRunning.data = 7;...
        | send(axis_isNotRunning)}
    (junction 2629) -> (junction 2628)
    (junction 2372) -> Axis_C2.DONE [order 1] : [RUN_idx == RUN_num_steps]
    Axis_C2.DONE -> (junction 2629)
  data: inp_data function_input; iPoints function_output; iP_dist function_input; inp_data function_input; whichAxis function_input; cV_init function_output; maxV function_input; iPoints function_input; cVec function_input; execVec function_output; iteratorStep function_input; whichAxis function_input; inp_data function_input; iPoints function_output; iP_dist function_input; inp_data function_input; center function_input; workspace function_input; kindOfAxis function_input; pointsForAxis function_output; num_registeredAxes local =0; num_collectedCVectors local =0; axis function_input; deltaS function_input; vel function_input; axis function_input; tPos function_input; tVel function_input; axis function_input; axis function_input; axis function_input; axis_is_moving local =0; currPos local =0; axis function_input; iP local size=[numAxes maxVectorLengths]; cVector_init local size=[1 maxVectorLengths]; PAR_isAxis constant double =1; PAR_maxVel constant double =0.12; axisHasSentCVector local =0; execVec local size=[4 maxVectorLengths] =1; RUN_idx local size=1 =0; currStepTimeLength local =0; RUN_num_steps local =0; MvmtPerf_accumulatedLagTime local =0; PAR_Bootstrap_deltaS constant double =1; FLAG_bootstrap_completed local =0; currCVector local size=[1 numAxes] =zeros(1,numAxes); currCVal local =0; currOverrideAdaptationFactor local =1; PAR_resetAxis_deltaS constant double =0.005; axis function_input; deltaS function_input; vel function_input; axis function_input; tPos function_input; tVel function_input; axis function_input; axis function_input; axis function_input; axis_is_moving local =0; currPos local =0; axis function_input; iP local size=[numAxes maxVectorLengths]; cVector_init local size=[1 maxVectorLengths]; PAR_isAxis constant double =2; PAR_maxVel constant double =0.12; axisHasSentCVector local =0; execVec local size=[4 maxVectorLengths] =1; RUN_idx local size=1 =0; currStepTimeLength local =0; RUN_num_steps local =0; MvmtPerf_accumulatedLagTime local =0; PAR_Bootstrap_deltaS constant double =1; FLAG_bootstrap_completed local =0; currCVector local size=[1 numAxes] =zeros(1,numAxes); currCVal local =0; currOverrideAdaptationFactor local =1; PAR_resetAxis_deltaS constant double =0.005; axis function_input; deltaS function_input; vel function_input; axis function_input; tPos function_input; tVel function_input; axis function_input; axis function_input; axis function_input; axis_is_moving local =0; currPos local =0; axis function_input; iP local size=[numAxes maxVectorLengths]; cVector_init local size=[1 maxVectorLengths]; PAR_isAxis constant double =3; PAR_maxVel constant double =0.05; axisHasSentCVector local =0; execVec local size=[4 maxVectorLengths] =1; RUN_idx local size=1 =0; currStepTimeLength local =0; RUN_num_steps local =0; MvmtPerf_accumulatedLagTime local =0; PAR_Bootstrap_deltaS constant double =1; FLAG_bootstrap_completed local =0; currCVector local size=[1 numAxes] =zeros(1,numAxes); currCVal local =0; currOverrideAdaptationFactor local =1; PAR_resetAxis_deltaS constant double =0.005; iP local size=[numAxes maxVectorLengths]; cVector_init local size=[1 maxVectorLengths]; PAR_isAxis constant double =4; PAR_maxVel constant double =100; axisHasSentCVector local =0; execVec local size=[4 maxVectorLengths] =1; RUN_idx local size=1 =0; currStepTimeLength local =0; RUN_num_steps local =0; MvmtPerf_accumulatedLagTime local =0; currCVector local size=[1 numAxes] =zeros(1,numAxes); currCVal local =0; currOverrideAdaptationFactor local =1; PAR_kindOfAxis constant double =6; FLAG_stopSim output =0; setP input; setP_dist input; registerAxis local; FLAG_canSend_cVector local =1; cVector_exchange local size=[1 maxVectorLengths]; cVector_sent local =1; cVectors local size=[numAxes maxVectorLengths] =0; FLAG_cVectors_complete local =0; PAR_execIteratorStepSize constant double =1; axis_ready local =0; num_readyAxes local =0; FLAG_allAxesReady local boolean =false; FLAG_doAkima local =0; axis_done local =0; num_doneAxes local =0; RUN_maxVel output size=[1 numAxes] =ones(1,numAxes); RUN_pos output size=[1 numAxes] =zeros(1,numAxes); RUN_startPos output size=[1 numAxes] =zeros(1,numAxes); RUN_time output size=[1 numAxes] =zeros(1,numAxes); RUN_vel output size=[1 numAxes] =zeros(1,numAxes); MvmtPerfEval_sendOwnVal parameter; GET_perfIndicator data_store_memory; MvmtPerfCoeff local =1; MvmtPerf local =1; RUN_MvmtPerfFeedback output size=[1 numAxes] =zeros(1,numAxes); MvmtPerfEval_collectVal parameter; Ts parameter; PAR_startPosReachedTol parameter; GET_istPos data_store_memory; VelOverride data_store_memory; PAR_numStepsAheadSmoothing parameter; FLAG_startButton data_store_memory; axis_isRunning local =0; num_runningAxes local =0; FLAG_stopButton data_store_memory; FLAG_resetAxis data_store_memory; FLAG_runContinuously data_store_memory; PAR_center_c2 parameter; PAR_workspace_c2 parameter; axis_isNotRunning local =0; FLAG_axesRunning data_store_memory; ff local =0; daten local =0
  function iPoints = DS_hermIntp(inp_data,iP_dist):
    | function iPoints = DS_hermIntp(inp_data,iP_dist)
    |  
    | 
    | euklid_abstand = vecnorm(diff(inp_data,1,2));
    | 
    | laufparam = cumsum(euklid_abstand);
    | laufparam = laufparam / max(laufparam);
    | laufparam = [0 laufparam];
    | 
    | 
    | anzahl_stuetzpunkte = 150;
    | anzahl_dim = size(inp_data,1);
    | iPoints = zeros(anzahl_dim,anzahl_stuetzpunkte);
    | 
    | for i=1:anzahl_dim
    |    
    |     iPoints(i,:) = pchip(laufparam,inp_data(i,:),linspace(0,1,anzahl_stuetzpunkte));
    |     
    | end
    | 
    | end
  function cV_init = DS_gen_Cvector_init(inp_data,whichAxis,maxV):
    | function cV_init = DS_gen_Cvector_init(inp_data,whichAxis,maxV)
    |  
    | safety_margin = 0.2; % max. Geschwindigkeit wird auf 80% der eigentlichen Fähigkeit der Achse festgelegt
    | 
    | wegdaten_raw = inp_data(whichAxis,:);
    | 
    | streckensegmente_raw = diff(wegdaten_raw);
    | 
    | 
    | zeitsegmente_raw = streckensegmente_raw ./ (maxV * (1 - safety_margin));
    | 
    | 
    | cV_init = abs(zeitsegmente_raw);
    | 
    | 
    | end
  function execVec = DS_find_Consensus(iPoints,cVec,iteratorStep,whichAxis):
    | function execVec = DS_find_Consensus(iPoints,cVec,iteratorStep,whichAxis)
    | 
    | cVector = max(cVec);
    | 
    | if(iteratorStep > 1)
    |    
    |     if(mod(size(iPoints,2)-1,iteratorStep) == 0)
    |         
    |         array_size = (size(iPoints,2) - 1) / iteratorStep;
    |         iPoints_relevant = zeros(1,array_size);
    |         
    |     else
    |        
    |         array_size = floor((size(iPoints,2) - 1) / iteratorStep) + 1;
    |         iPoints_relevant = zeros(1,array_size);
    |         
    |     end
    |     
    |     
    |     iPoints_relevant = iPoints(whichAxis,1:iteratorStep:end);
    |     
    |     % Neue Zeitabschnitte berechnen
    |     for ii=1:array_size-1
    |        
    |         currIdx = ((ii-1) * iteratorStep) + 1;
    |         zP = cVec(1,currIdx : currIdx + iteratorStep);
    |         
    |         zeitabschnitte = sum(zP);
    |         
    |     end
    | 
    |     
    | else
    |    
    |     iPoints_relevant = iPoints(whichAxis,:);
    | 
    |     
    | end
    | 
    |     wegabschnitte = diff(iPoints_relevant(1,:));
    |     zeitabschnitte = cVector;
    |     absolute_zeitpunkte = cumsum(zeitabschnitte);
    |     
    |     geschwindigkeiten = abs(wegabschnitte ./ zeitabschnitte);
    |     
    |     execVec = [iPoints_relevant(2:end);...
    |         geschwindigkeiten;...
    |         zeitabschnitte;...
    |         absolute_zeitpunkte];
    | 
    | 
    | 
    | end
  function iPoints = DS_hermIntp_old(inp_data,iP_dist):
    | function iPoints = DS_hermIntp_old(inp_data,iP_dist)
    |  
    | x = inp_data(1,:);
    | y = inp_data(2,:);
    | 
    | x_zwischenpunkte = (x(1):iP_dist:x(end));
    | 
    | y_interpoliert = pchip(x,y,x_zwischenpunkte);
    | 
    | iPoints = [x_zwischenpunkte; y_interpoliert];
    | 
    | 
    | end
  function pointsForAxis  = PS_gen_Points_Axis(inp_data,center,workspace,kindOfAxis):
    | function pointsForAxis  = PS_gen_Points_Axis(inp_data,center,workspace,kindOfAxis)
    |  
    | coder.extrinsic('PS_Hiwin_getPos');
    | 
    | mX = center(1);
    | mY = center(2);
    | mZ = center(3);
    | wsXWide = workspace(1);
    | wsYWide = workspace(2);
    | wsZWide = workspace(3);
    | wsRadiusIn = workspace(4);
    | wsRadiusOut = workspace(5);
    | radius = (workspace(4)+workspace(5))/2;
    | inp_data(2,:) = -inp_data(2,:)+2*mY;
    | 
    | outputPoints = zeros(1,length(inp_data));
    | 
    | switch kindOfAxis
    |     case 1
    |         %X2 Achse
    |         for i=1: (length(inp_data))
    |             if (inp_data(1,i) <= mX + wsXWide/2) && (inp_data(1,i) >= mX - wsXWide/2) &&...
    |                     (inp_data(2,i) <= mY + wsYWide/2) && (inp_data(2,i) >= mY - wsYWide/2) &&...
    |                     (inp_data(3,i) <= mZ + wsZWide/2) && (inp_data(3,i) >= mZ - wsZWide/2)
    |                 outputPoints(i) = inp_data(1,i);
    |             else
    |                 if i>1
    |                     outputPoints(i) = outputPoints(i-1);
    |                 else
    |                     outputPoints(i) = mX - wsXWide/2;
    |                 end
    |             end
    |         end
    |     case 2
    |         %Y2 Achse
    |     case 3
    |         %Z2 Achse
    |     case 4
    |         %A Achse
    |     case 5
    |         %B Achse
    |     case 6
    |         % C Achse
    |         zeroDegreePoint = [mX-radius;mY];
    |         zeroDegreeVec = [zeroDegreePoint(1)-mX; zeroDegreePoint(2)-mY];
    |         for i=1: (length(inp_data))
    |             % Prüfung ob Bahnkurve durch den Arbeitsraum verläuft
    |             if (inp_data(3,i) <= mZ + wsZWide/2) && (inp_data(3,i) >= mZ - wsZWide/2) &&...
    |                     (wsRadiusIn <= sqrt((inp_data(1,i)-mX)^2+(inp_data(2,i)-mY)^2)) &&...
    |                     (wsRadiusOut >= sqrt((inp_data(1,i)-mX)^2+(inp_data(2,i)-mY)^2))
    |                 % Bestimmung des absoluten Winkels
    |                 pos = [inp_data(1,i)-mX; inp_data(2,i)-mY];
    |                 alpha = acos(dot(zeroDegreeVec,pos)/(norm(zeroDegreeVec)*norm(pos)))*180/pi;
    |                 % Berücksichtigung Richtungsumkehr
    |                 if inp_data(2,i)-mY < 0
    |                     alpha = 360 - alpha;
    |                 end
    |                 % Berechnung des Zielwinkels
    |                 if i>1
    |                     outputPoints(i) = outputPoints(i-1) + mod((alpha - outputPoints(i-1)),360/6);
    |                 else
    |                     outputPoints(i) = mod(alpha,360/6);
    |                 end
    |             else
    |                 if i>1
    |                     outputPoints(i) = outputPoints(i-1);
    |                 else
    |                     outputPoints(i) = PS_Hiwin_getPos();
    |                 end
    |             end
    |         end
    | end
    | pointsForAxis = outputPoints;
    | end
  function moveRel(axis,deltaS,vel):
    | function moveRel(axis,deltaS,vel)
    | 
    | coder.extrinsic('V_2_x_moveRel');
    | V_2_x_moveRel(axis,deltaS,vel);
    | 
    | 
    | end
  function goToPos(axis,tPos,tVel):
    | function goToPos(axis,tPos,tVel)
    | 
    | coder.extrinsic('V_2_x_goToPos');
    | V_2_x_goToPos(axis,tPos,tVel);
    | 
    | 
    | end
  function StopAxis(axis):
    | function StopAxis(axis)
    | 
    | coder.extrinsic('V_2_x_STOP');
    | V_2_x_STOP(axis);
    | 
    | 
    | end
  function ResetAxis(axis):
    | function ResetAxis(axis)
    | 
    | coder.extrinsic('PS_ResetAxis');
    | PS_ResetAxis(axis);
    | end
  function jogAxis(axis):
    | function jogAxis(axis)
    | 
    | coder.extrinsic('V_2_x_Jogging');
    | V_2_x_Jogging(axis);
    | 
    | 
    | end
  function ResetAxis(axis):
    | function ResetAxis(axis)
    | 
    | coder.extrinsic('PS_ResetAxis');
    | PS_ResetAxis(axis);
    | end
  function moveRel(axis,deltaS,vel):
    | function moveRel(axis,deltaS,vel)
    | 
    | coder.extrinsic('V_2_x_moveRel');
    | V_2_x_moveRel(axis,deltaS,vel);
    | 
    | 
    | end
  function goToPos(axis,tPos,tVel):
    | function goToPos(axis,tPos,tVel)
    | 
    | coder.extrinsic('V_2_x_goToPos');
    | V_2_x_goToPos(axis,tPos,tVel);
    | 
    | 
    | end
  function StopAxis(axis):
    | function StopAxis(axis)
    | 
    | coder.extrinsic('V_2_x_STOP');
    | V_2_x_STOP(axis);
    | 
    | 
    | end
  function ResetAxis(axis):
    | function ResetAxis(axis)
    | 
    | coder.extrinsic('PS_ResetAxis');
    | PS_ResetAxis(axis);
    | end
  function jogAxis(axis):
    | function jogAxis(axis)
    | 
    | coder.extrinsic('V_2_x_Jogging');
    | V_2_x_Jogging(axis);
    | 
    | 
    | end
  function ResetAxis(axis):
    | function ResetAxis(axis)
    | 
    | coder.extrinsic('PS_ResetAxis');
    | PS_ResetAxis(axis);
    | end
  function moveRel(axis,deltaS,vel):
    | function moveRel(axis,deltaS,vel)
    | 
    | coder.extrinsic('V_2_x_moveRel');
    | V_2_x_moveRel(axis,deltaS,vel);
    | 
    | 
    | end
  function goToPos(axis,tPos,tVel):
    | function goToPos(axis,tPos,tVel)
    | 
    | coder.extrinsic('V_2_x_goToPos');
    | V_2_x_goToPos(axis,tPos,tVel);
    | 
    | 
    | end
  function StopAxis(axis):
    | function StopAxis(axis)
    | 
    | coder.extrinsic('V_2_x_STOP');
    | V_2_x_STOP(axis);
    | 
    | 
    | end
  function ResetAxis(axis):
    | function ResetAxis(axis)
    | 
    | coder.extrinsic('PS_ResetAxis');
    | PS_ResetAxis(axis);
    | end
  function jogAxis(axis):
    | function jogAxis(axis)
    | 
    | coder.extrinsic('V_2_x_Jogging');
    | V_2_x_Jogging(axis);
    | 
    | 
    | end
  function ResetAxis(axis):
    | function ResetAxis(axis)
    | 
    | coder.extrinsic('PS_ResetAxis');
    | PS_ResetAxis(axis);
    | end
  function homingDauerlauf:
    | function homingDauerlauf
    | 
    | coder.extrinsic('PS_Hiwin_homingDauerlauf');
    | PS_Hiwin_homingDauerlauf;
    | end

== stateflow chart DS_distrIntp_4_0_realaxes/Achse Y/Achsgeschwindigkeit ==
  state new_measurement
    entry:
    if(oldTimeStamp) ~= 0
    delta_s = abs(Pos - oldPos);
    delta_t = TimeStamp - oldTimeStamp;
    velocity = delta_s / (delta_t / 1000);
    if sollGeschw ~= 0
    velocity_norm = velocity / (maxVelocity*0.8);
    else
    velocity_norm = 0;
    end
    end
  state Wait_for_new_measurement
    entry:
    oldPos = Pos;
    oldTimeStamp = TimeStamp;
  (default) -> Wait_for_new_measurement
  Wait_for_new_measurement -> new_measurement : [hasChanged(Pos) &&...
      |  hasChanged(TimeStamp)]
  new_measurement -> Wait_for_new_measurement
  data: Pos input; TimeStamp input; velocity output; delta_s local; delta_t local; oldPos local; oldTimeStamp local; velocity_norm output =0; maxVelocity input; sollGeschw input
